simulink model "c"  (R2020a)
settings: Solver=VariableStepAuto  StartTime=0.0  StopTime=10.0  RelTol=1e-3
settings Model: OrderedModelArguments=off  Creator=mahmo  LastModifiedBy=mahmo

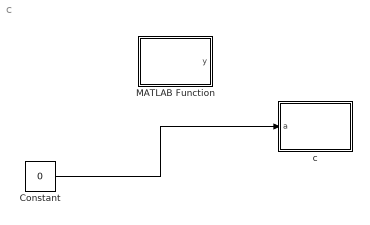
== system c ==
  Constant : Constant  Value=0
  MATLAB Function : MATLAB Function  TreatAsAtomicUnit=on
  c : MATLAB Function  TreatAsAtomicUnit=on
  wires:
  Constant/1 -> c/1(a)

== matlab function c/c ==
  data: a input
function c(a)
global b
writeDigitalPin(b,'D13',a);

== matlab function c/MATLAB Function ==
  data: y output
function y = fcn()

y =arduino('COM3','Uno','libraries','RotaryEncoder');
